simulink model "UDP_reader"  (R2021b)
settings: Solver=VariableStepAuto  StartTime=0.0  StopTime=inf  RelTol=1e-3
undefined symbols (not defined in the file): f
libraries: instrumentlib x1
settings Model: Creator=Titanium  LastModifiedBy=Titanium

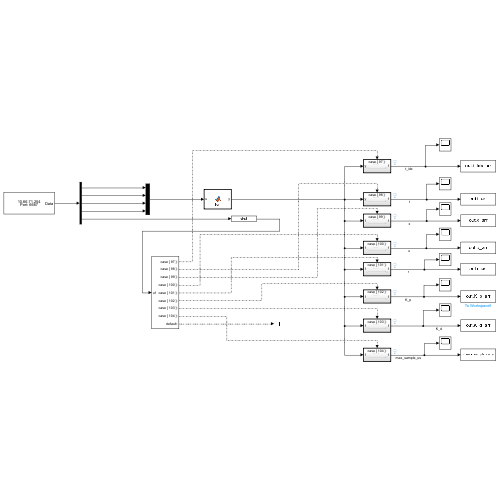
[thumbnail: Simulink's stored preview of the top-level diagram]
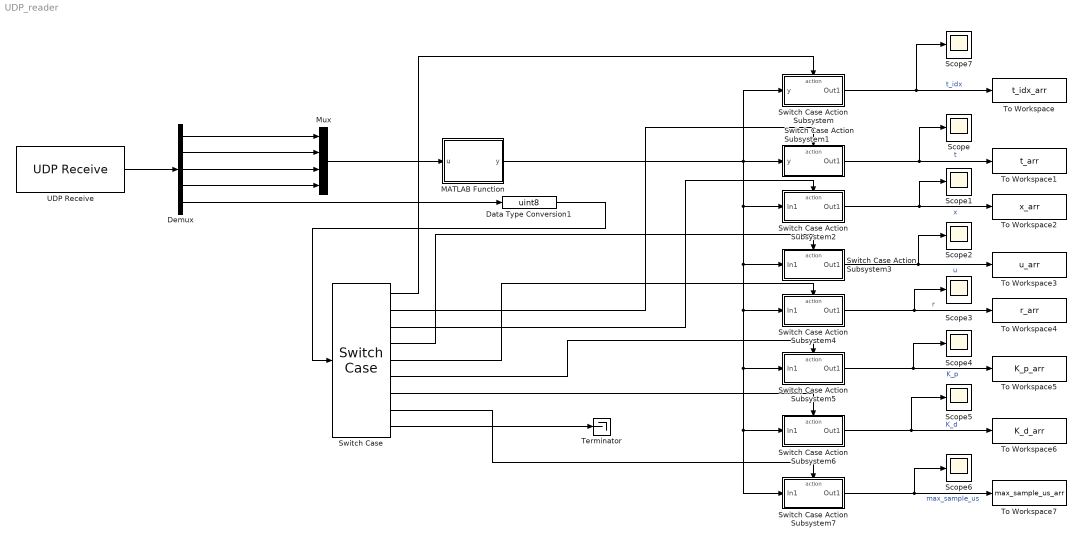
== system UDP_reader ==
  Data Type Conversion1 : DataTypeConversion  OutDataTypeStr=uint8
  Demux : Demux  Outputs=5
  MATLAB Function : MATLAB Function  TreatAsAtomicUnit=on
  Mux : Mux
  Scope{,1..7} (8 alike) : Scope
  Switch Case : SwitchCase  CaseConditions={97, 98, 99, 100, 101, 102, 103, 104}
  Switch Case Action Subsystem : Subsystem  TreatAsAtomicUnit=on
  Switch Case Action Subsystem1 : Subsystem  TreatAsAtomicUnit=on
  Switch Case Action Subsystem2 : Subsystem  TreatAsAtomicUnit=on
  Switch Case Action Subsystem3 : Subsystem  TreatAsAtomicUnit=on
  Switch Case Action Subsystem4 : Subsystem  TreatAsAtomicUnit=on
  Switch Case Action Subsystem5 : Subsystem  TreatAsAtomicUnit=on
  Switch Case Action Subsystem6 : Subsystem  TreatAsAtomicUnit=on
  Switch Case Action Subsystem7 : Subsystem  TreatAsAtomicUnit=on
  Terminator : Terminator
  To Workspace : ToWorkspace  VariableName=t_idx_arr  SampleTime=-1
  To Workspace1 : ToWorkspace  VariableName=t_arr  SampleTime=-1
  To Workspace2 : ToWorkspace  VariableName=x_arr  SampleTime=-1
  To Workspace3 : ToWorkspace  VariableName=u_arr  SampleTime=-1
  To Workspace4 : ToWorkspace  VariableName=r_arr  SampleTime=-1
  To Workspace5 : ToWorkspace  VariableName=K_p_arr  SampleTime=-1
  To Workspace6 : ToWorkspace  VariableName=K_d_arr  SampleTime=-1
  To Workspace7 : ToWorkspace  VariableName=max_sample_us_arr  SampleTime=-1
  UDP Receive : instrumentlib/UDP Receive  Host=10.66.203.90  Port=6667  LocalPort=6667  EnablePortSharing=off  GetLatestData=off  DataSize="[5  1]"  DataType=uint8  ASCIIFormatting=%f,  Terminator=LF  ByteOrder=BigEndian  EnableBlockingMode=on  Timeout=10  SampleTime=0.01  LocalAddress=10.66.71.254
  wires:
  UDP Receive/1 -> Demux/1
  Demux/5 -> Data Type Conversion1/1
  Data Type Conversion1/1 -> Switch Case/1
  Switch Case Action Subsystem/1(Out1) -> Scope7/1, To Workspace/1  "t_idx"
  Switch Case Action Subsystem1/1(Out1) -> Scope/1, To Workspace1/1  "t"
  Switch Case Action Subsystem2/1(Out1) -> Scope1/1, To Workspace2/1  "x"
  Switch Case Action Subsystem3/1(Out1) -> Scope2/1, To Workspace3/1  "u"
  Switch Case Action Subsystem4/1(Out1) -> Scope3/1, To Workspace4/1  "r"
  Switch Case Action Subsystem5/1(Out1) -> Scope4/1, To Workspace5/1  "K_p"
  Switch Case Action Subsystem6/1(Out1) -> Scope5/1, To Workspace6/1  "K_d"
  Switch Case Action Subsystem7/1(Out1) -> Scope6/1, To Workspace7/1  "max_sample_us"
  Switch Case/9 -> Terminator/1
  Switch Case/8 -> Switch Case Action Subsystem7/Action
  Switch Case/7 -> Switch Case Action Subsystem6/Action
  Switch Case/6 -> Switch Case Action Subsystem5/Action
  Switch Case/5 -> Switch Case Action Subsystem4/Action
  Switch Case/4 -> Switch Case Action Subsystem3/Action
  Switch Case/3 -> Switch Case Action Subsystem2/Action
  Switch Case/2 -> Switch Case Action Subsystem1/Action
  Switch Case/1 -> Switch Case Action Subsystem/Action
  Demux/1 -> Mux/1
  Demux/2 -> Mux/2
  Demux/3 -> Mux/3
  Demux/4 -> Mux/4
  MATLAB Function/1(y) -> Switch Case Action Subsystem1/1(y), Switch Case Action Subsystem/1(y), Switch Case Action Subsystem2/1(In1), Switch Case Action Subsystem3/1(In1), Switch Case Action Subsystem7/1(In1), Switch Case Action Subsystem6/1(In1), Switch Case Action Subsystem5/1(In1), Switch Case Action Subsystem4/1(In1)
  Mux/1 -> MATLAB Function/1(u)

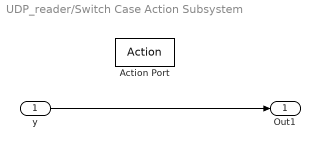
== system UDP_reader/Switch Case Action Subsystem ==
  y : Inport
  Action Port : ActionPort  ActionPortLabel=case [ 97 ]:
  Out1 : Outport
  wires:
  y/1 -> Out1/1

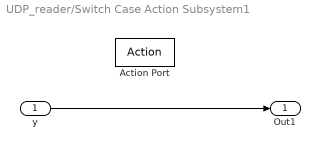
== system UDP_reader/Switch Case Action Subsystem1 ==
  y : Inport
  Action Port : ActionPort  ActionPortLabel=case [ 98 ]:
  Out1 : Outport
  wires:
  y/1 -> Out1/1

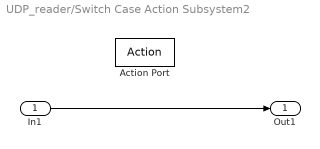
== system UDP_reader/Switch Case Action Subsystem2 ==
  In1 : Inport
  Action Port : ActionPort  ActionPortLabel=case [ 99 ]:
  Out1 : Outport
  wires:
  In1/1 -> Out1/1

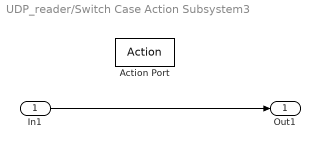
== system UDP_reader/Switch Case Action Subsystem3 ==
  In1 : Inport
  Action Port : ActionPort  ActionPortLabel=case [ 100 ]:
  Out1 : Outport
  wires:
  In1/1 -> Out1/1

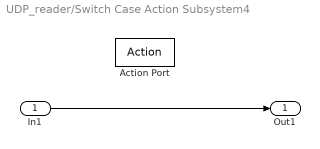
== system UDP_reader/Switch Case Action Subsystem4 ==
  In1 : Inport
  Action Port : ActionPort  ActionPortLabel=case [ 101 ]:
  Out1 : Outport
  wires:
  In1/1 -> Out1/1

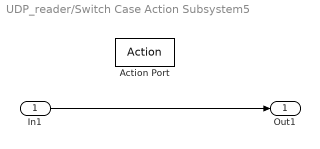
== system UDP_reader/Switch Case Action Subsystem5 ==
  In1 : Inport
  Action Port : ActionPort  ActionPortLabel=case [ 102 ]:
  Out1 : Outport
  wires:
  In1/1 -> Out1/1

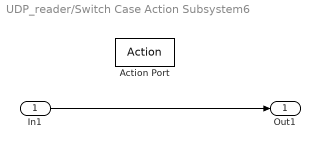
== system UDP_reader/Switch Case Action Subsystem6 ==
  In1 : Inport
  Action Port : ActionPort  ActionPortLabel=case [ 103 ]:
  Out1 : Outport
  wires:
  In1/1 -> Out1/1

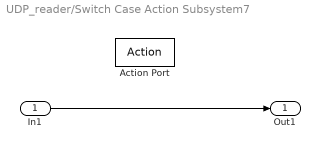
== system UDP_reader/Switch Case Action Subsystem7 ==
  In1 : Inport
  Action Port : ActionPort  ActionPortLabel=case [ 104 ]:
  Out1 : Outport
  wires:
  In1/1 -> Out1/1

== matlab function UDP_reader/MATLAB Function ==
  data: u input uint8 size=[4 1]; y output single size=1
function y = fcn(u)

y = single(typecast(uint8([u(1) u(2) u(3) u(4)]), 'single'));
